simulink model "LQG_Reference_gain"  (R2022b)
settings: Solver=VariableStepAuto  StartTime=0.0  StopTime=60  RelTol=1e-3
values from neighbouring files (symbols this model uses):
  Ad = [0.401010357696 0.207607414378 0.0585143980091 -782.832786661 342.529887341 0.596372065474 0.774865707155 0.568579797376 773.747483889 -370.95887721 0.00261757683024 0.0175268784671 ... (25 elements, 5x5)]    [A_d.mat]    (also in ref.m = expm(Av*Ts))
  Bd = [0.00315440131404  0.000285742610066; 0.000159453102519  0.00321146251052; 2.85742610066e-05  0.316758560203; 4.4993079134  1.30878841512; 0.585143980091  8.76343923355]    [B_d.mat]    (also in ref.m = double(int(exp_At,t,0,Ts)*Bv))
  C1 = [0  1  0  0  0; 0  0  0  0  1]    [C.mat]    (also in ref.m = jacobian(x(:,1), [phi2(1);w2(1)]).')
  D_1 = [0  0; 0  0]    [D.mat]
  K = dlqr(Ad,Bd,Qx,Qu,N)    [Assignment3.m]
  Kr1 = diag(Kr1)*1e-14    [Assignment3.m]
undefined symbols (not defined in the file or in its folder): L
settings Model: Creator=aksha  LastModifiedBy=aksha

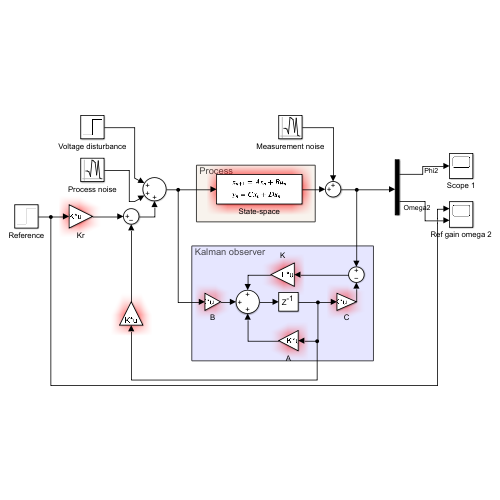
[thumbnail: Simulink's stored preview of the top-level diagram]
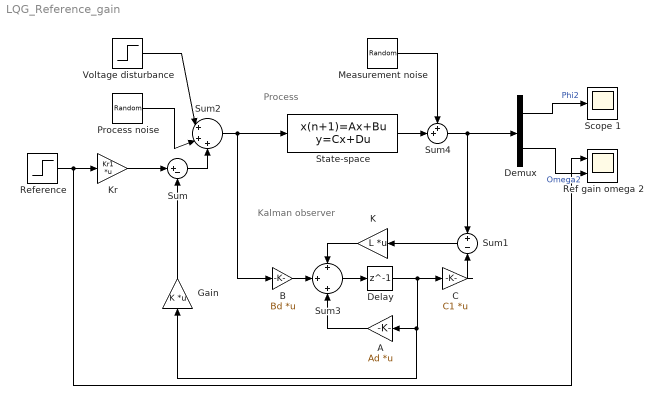
== system LQG_Reference_gain ==
  note: Process
  note: Kalman observer
  A : Gain  Gain=Ad  Multiplication=Matrix(K*u)
  B : Gain  Gain=Bd  Multiplication=Matrix(K*u)
  C : Gain  Gain=C1  Multiplication=Matrix(K*u)
  Delay : Delay  DelayLength=1
  Demux : Demux  Outputs=2
  Gain : Gain  Gain=K  Multiplication=Matrix(K*u)
  K : Gain  Gain=L  Multiplication=Matrix(K*u)
  Kr : Gain  Gain=Kr1  Multiplication=Matrix(K*u)
  Measurement noise : RandomNumber  Variance=[(0.02/3)^2 ; (0.01/3)^2]  SampleTime=0.1
  Process noise : RandomNumber  Variance=[(0.3/3)^2; (0.1/3)^2]  SampleTime=0.1
  Ref gain omega 2 : Scope  NumInputPorts=2
  Reference : Step  Time=10  Before=10  After=100  SampleTime=0
  Scope 1 : Scope
  State-space : DiscreteStateSpace  A=Ad  B=Bd  C=C1  D=D_1  SampleTime=-1
  Sum : Sum  Inputs=|+-
  Sum1 : Sum  Inputs=+|-
  Sum2 : Sum  Inputs=|+++
  Sum3 : Sum  Inputs=+|+|+
  Sum4 : Sum  Inputs=++|
  Voltage disturbance : Step  Time=5  SampleTime=0
  wires:
  B/1 -> Sum3/2
  Kr/1 -> Sum/1
  Reference/1 -> Ref gain omega 2/1, Kr/1
  Demux/1 -> Scope 1/1  "Phi2"
  Gain/1 -> Sum/2
  Sum3/1 -> Delay/1
  K/1 -> Sum3/1
  A/1 -> Sum3/3
  Delay/1 -> C/1, Gain/1, A/1
  C/1 -> Sum1/2
  Sum1/1 -> K/1
  Sum/1 -> Sum2/3
  Sum2/1 -> State-space/1, B/1
  Sum4/1 -> Demux/1, Sum1/1
  State-space/1 -> Sum4/2
  Measurement noise/1 -> Sum4/1
  Process noise/1 -> Sum2/2
  Voltage disturbance/1 -> Sum2/1
  Demux/2 -> Ref gain omega 2/2  "Omega2"
